simulink model "for_iterator_test"  (Simulink 8.4)
settings: Solver=VariableStepDiscrete  StartTime=0.0  StopTime=1  MaxStep=1  RelTol=1e-3
settings Model: Creator=arnaud  LastModifiedBy=arnaud
settings DataIOCC: SaveFormat=Structure  SignalLoggingSaveFormat=Dataset
settings OptimizationCC: ExpressionDepthLimit=128
settings DebuggingCC: UnderspecifiedInitializationDetection=Simplified  MergeDetectMultiDrivingBlocksExec=error  FcnCallInpInsideContextMsg=EnableAllAsError  StateNameClashWarn=none
settings GRTTargetCC: CombineOutputUpdateFcns=on  GRTInterface=off

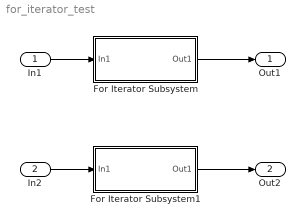
== system for_iterator_test ==
  In1 : Inport
  In2 : Inport  Port=2
  For Iterator Subsystem : Subsystem  TreatAsAtomicUnit=on
  For Iterator Subsystem1 : Subsystem  TreatAsAtomicUnit=on
  Out1 : Outport
  Out2 : Outport  Port=2
  wires:
  For Iterator Subsystem/1(Out1) -> Out1/1
  In1/1 -> For Iterator Subsystem/1(In1)
  For Iterator Subsystem1/1(Out1) -> Out2/1
  In2/1 -> For Iterator Subsystem1/1(In1)

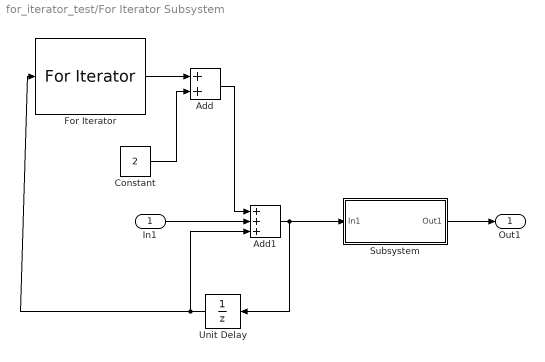
== system for_iterator_test/For Iterator Subsystem ==
  In1 : Inport
  Add : Sum
  Add1 : Sum  Inputs=+++
  Constant : Constant  Value=2  OutDataTypeStr=int32
  For Iterator : ForIterator  ResetStates=reset  ExternalIncrement=on
  Subsystem : Subsystem  TreatAsAtomicUnit=on
  Unit Delay : UnitDelay  InitialCondition=2  SampleTime=-1
  Out1 : Outport
  wires:
  Constant/1 -> Add/2
  Add1/1 -> Unit Delay/1, Subsystem/1(In1)
  Unit Delay/1 -> For Iterator/1, Add1/3
  Subsystem/1(Out1) -> Out1/1
  For Iterator/1 -> Add/1
  In1/1 -> Add1/2
  Add/1 -> Add1/1

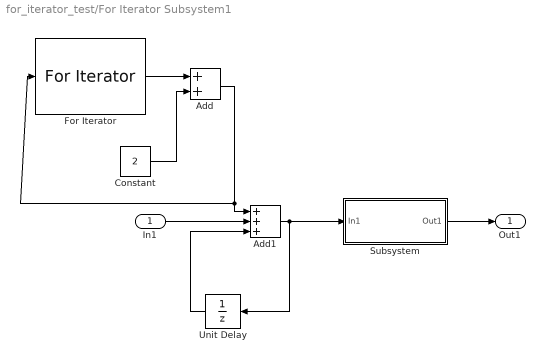
== system for_iterator_test/For Iterator Subsystem1 ==
  In1 : Inport  PortDimensions=3
  Add : Sum
  Add1 : Sum  Inputs=+++
  Constant : Constant  Value=2  OutDataTypeStr=int32
  For Iterator : ForIterator  ResetStates=reset  ExternalIncrement=on  IndexMode=Zero-based
  Subsystem : Subsystem  TreatAsAtomicUnit=on
  Unit Delay : UnitDelay  InitialCondition=2  SampleTime=-1
  Out1 : Outport
  wires:
  Constant/1 -> Add/2
  Add1/1 -> Unit Delay/1, Subsystem/1(In1)
  Unit Delay/1 -> Add1/3
  Subsystem/1(Out1) -> Out1/1
  For Iterator/1 -> Add/1
  In1/1 -> Add1/2
  Add/1 -> For Iterator/1, Add1/1

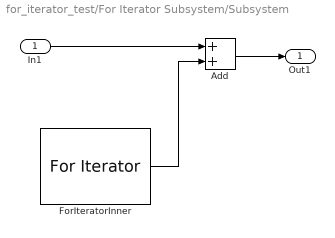
== system for_iterator_test/For Iterator Subsystem/Subsystem ==
  In1 : Inport
  Add : Sum
  ForIteratorInner : ForIterator  IterationLimit=4  IterationVariableDataType=double
  Out1 : Outport
  wires:
  In1/1 -> Add/1
  ForIteratorInner/1 -> Add/2
  Add/1 -> Out1/1

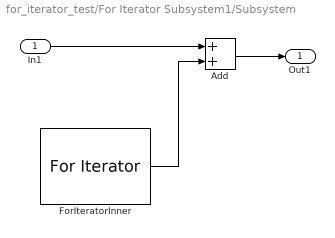
== system for_iterator_test/For Iterator Subsystem1/Subsystem ==
  In1 : Inport
  Add : Sum
  ForIteratorInner : ForIterator  ResetStates=reset  IterationLimit=4  IndexMode=Zero-based  IterationVariableDataType=double
  Out1 : Outport
  wires:
  In1/1 -> Add/1
  ForIteratorInner/1 -> Add/2
  Add/1 -> Out1/1
